simulink model "HB"  (R2023a)
settings: Solver=VariableStepAuto  StartTime=0.0  StopTime=0.1  RelTol=1e-3
undefined symbols (not defined in the file): plecs, Ts
libraries: plecslib x5
settings Model: Creator=lokit  LastModifiedBy=lokit

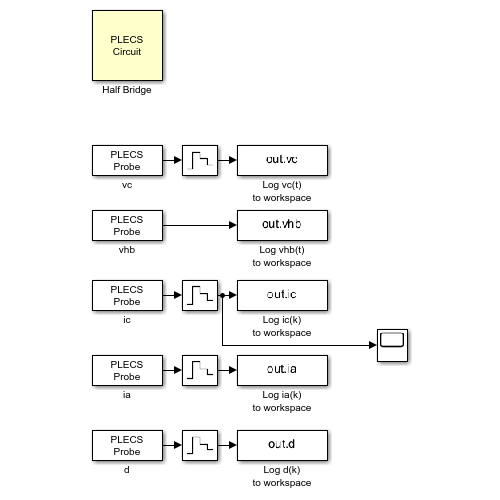
[thumbnail: Simulink's stored preview of the top-level diagram]
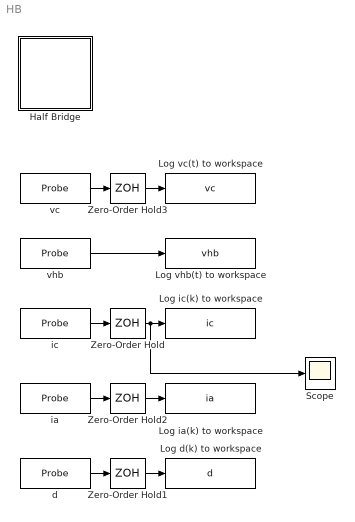
== system HB ==
  Half Bridge : Subsystem  LoadFcn=plecs('sl', 200);  InitFcn=plecs('sl', 214);  StartFcn=plecs('sl', 208);  StopFcn=plecs('sl', 209);  mask(PlecsCircuit){PLECSData=<binary blob, 5296 chars, not shown>}
      mask prompts: PLECSData "PLECS Data (Do not delete or modify!)"
      mask init:
      | % PLACE CUSTOM INITIALIZATIONS ABOVE
      | % DO NOT REMOVE
      | plecs('sl', 215);
      | % DO NOT REMOVE
      settings: CopyFcn=plecs('sl', 203);  DeleteFcn=plecs('sl', 205);  UndoDeleteFcn=plecs('sl', 206);  PreSaveFcn=plecs('sl', 211);  PostSaveFcn=plecs('sl', 201);  NameChangeFcn=plecs('sl', 210);  DestroyFcn=plecs('sl', 207);  PreCopyFcn=plecs('sl', 216);  OpenFcn=plecs('sl', 202);  ErrorFcn=plerrorfcn
      mask Help: eval('plecs(''help'', ''qthelp:///creatingacircuit.html'')')
      mask Display: disp('PLECS\nCircuit')
  Log d(k) to workspace : ToWorkspace  VariableName=d  SaveFormat=Timeseries  SampleTime=-1
  Log ia(k) to workspace : ToWorkspace  VariableName=ia  SaveFormat=Timeseries  SampleTime=-1
  Log ic(k) to workspace : ToWorkspace  VariableName=ic  SaveFormat=Timeseries  SampleTime=-1
  Log vc(t) to workspace : ToWorkspace  VariableName=vc  SaveFormat=Timeseries  SampleTime=-1
  Log vhb(t) to workspace : ToWorkspace  VariableName=vhb  SaveFormat=Timeseries  SampleTime=-1
  Scope : Scope
  Zero-Order Hold{,1..3} (4 alike) : ZeroOrderHold  SampleTime=Ts
  d : plecslib/Probe  tagno=3
      settings: SourceProductName=PLECS
  ia : plecslib/Probe  tagno=4
      settings: SourceProductName=PLECS
  ic : plecslib/Probe  tagno=2
      settings: SourceProductName=PLECS
  vc : plecslib/Probe  tagno=1
      settings: SourceProductName=PLECS
  vhb : plecslib/Probe  tagno=5
      settings: SourceProductName=PLECS
  wires:
  ic/1 -> Zero-Order Hold/1
  d/1 -> Zero-Order Hold1/1
  Zero-Order Hold2/1 -> Log ia(k) to workspace/1
  ia/1 -> Zero-Order Hold2/1
  vhb/1 -> Log vhb(t) to workspace/1
  vc/1 -> Zero-Order Hold3/1
  Zero-Order Hold3/1 -> Log vc(t) to workspace/1
  Zero-Order Hold/1 -> Scope/1, Log ic(k) to workspace/1
  Zero-Order Hold1/1 -> Log d(k) to workspace/1

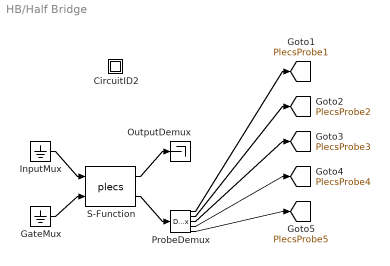
== system HB/Half Bridge ==
  " CircuitID2 " : Subsystem
  " GateMux " : Ground
  " InputMux " : Ground
  " OutputDemux " : Terminator
  " ProbeDemux " : Demux  Outputs=[ 1 1 1 1 1 ]
  " S-Function " : S-Function  FunctionName=plecs  SFunctionDeploymentMode=off  EnableBusSupport=off
  tag scope: PlecsProbe1=global, PlecsProbe2=global, PlecsProbe3=global, PlecsProbe4=global, PlecsProbe5=global
  wires:
  " InputMux "/1 -> " S-Function "/1
  " GateMux "/1 -> " S-Function "/2
  " S-Function "/1 -> " OutputDemux "/1
  " S-Function "/2 -> " ProbeDemux "/1
  " ProbeDemux "/1 -> [PlecsProbe1]
  " ProbeDemux "/2 -> [PlecsProbe2]
  " ProbeDemux "/3 -> [PlecsProbe3]
  " ProbeDemux "/4 -> [PlecsProbe4]
  " ProbeDemux "/5 -> [PlecsProbe5]

== system HB/Half Bridge/ CircuitID2  ==
